simulink model "remoteMicrogrid"  (R2023a)
settings: Solver=FixedStepDiscrete  StartTime=0.0  StopTime=8  FixedStep=Ts  RelTol=1e-3
PreLoadFcn:
  | remoteMicrogridInputData
undefined symbols (not defined in the file): BESS, ControlRoom, DiscIntNeverNeededParam, Grid, Load, Machine, Microgrid, PV, T_on, Ts
libraries: ee_lib x46, eeGeneralControl x35, nesl_utility_internal x25, simulink x24, nesl_utility x20, fl_lib x17, slpidlib x12, eeTransforms x5, eeRmsMeasurement x4, eeTotalHarmonicDistorsion x4, eeSinusoidalMeasurement x3, batteryecm_lib x2
(part 2 of 5)

== system remoteMicrogrid/Diesel Substation, BESS, & Microgrid Controller/Diesel Generator ==
  AVR and Exciter : Subsystem
  "Governor and Prime Mover " : Subsystem  mask(Governor and Prime Mover){pu_speed_reference=Machine.SpeedReference, droop_percentage=Machine.Droop, pu_load_reference_setpoint=Machine.LoadReference, T_G=Machine.TimeConstandGovernor, T_CH=Machine.TimeConstantPrimeMover, base_torque=Machine.BaseTorque, pu_torque0=Machine.InitialTorque}
      mask prompts: pu_speed_reference "Speed reference, (pu)"; droop_percentage "Percentage droop, (%)"; pu_load_reference_setpoint "Load reference setpoint, (pu)"; T_G "Time constant of governor, (s)"; T_CH "Time constant of main inlet volumes and steam chest, (s)"; base_torque "Base torque, (N*m)"; pu_torque0 "Initial torque, (pu)"
      mask help:
      | Implements a synchronous machine governor and prime mover. The prime mover is a non-reheat steam turbine.
      |
      | The input to the block is a per-unit synchronous machine measurement vector.
      |
      | R and C are mechanical rotational ports.
  Machine Inertia : ee_lib/Electromechanical/Mechanical/Machine Inertia  SRated=Grid.DieselRatedPower V*A  FRated=Grid.Frequency Hz  nPolePairs=1  inertia_option=1  J=Machine.Inertia kg*m^2  H=3.525 s*W/V/A  damper_option=2  D=39.0509 N*m/(rad/s)  pu_D=0.01  initialization_option=2  fMechanical0=60 Hz  fElectrical0=Grid.Frequency Hz
      settings: InternalSimscapePortConfiguration="{\"Bottom\":[],\"Left\":[{\"id\":\"R\",\"label\":\"R\",\"type\":\"foundation.mechanical.rotational.rotational\"}],\"Right\":[],\"Top\":[]}"
  Rotational Friction : fl_lib/Mechanical/Rotational Elements/Rotational Friction  brkwy_trq=1.1 N*m  brkwy_vel=0.1 rad/s  Col_trq=0.05 N*m  visc_coef=0.001 N*m*s/rad  w_specify=off  w_priority=None  w=0 rad/s  w_nominal_specify=off  w_nominal_unit=rad/s  w_nominal_value=1  t_specify=off  t_priority=None  t=0 N*m  t_nominal_specify=off  t_nominal_unit=N*m  t_nominal_value=1
  Synchronous Machine Round Rotor : ee_lib/Electromechanical/Synchronous/Synchronous Machine Round Rotor  port_option=ee.enum.threePhasePort.composite  SRated=Grid.DieselRatedPower A*V  VRated=Grid.Voltage V  FRated=Grid.Frequency Hz  nPolePairs=1  param_option=ee.enum.sm.parameterization.standard  fieldCircuitParameterization_option=ee.enum.sm.fieldparameterization.current  baseEfd=92.95 V  baseIfd=1300 A  zero_sequence=ee.enum.park.zerosequence.include  axes_param=ee.enum.rotorangle.daxis  Ladu=1.66  Laqu=1.61  L0=0.15  Ll=0.05  Ra=0.03  Lfd=0.165  Rfd=0.0006  L1d=0.1713  R1d=0.0284  L1q=0.7252  R1q=0.00619  L2q=0.125  R2q=0.02368  Xl=0.05  Xd=1.72  Xq=0.79  X0=0.06  Xdd=0.13  Xqd=0.17  Xddd=0.09  Xqdd=0.12  d_option=ee.enum.circuit.open  Td0d=0.75 s  Tdd=0.03 s  Td0dd=0.03 s  Tddd=0.008 s  q_option=ee.enum.circuit.open  Tq0d=0.6 s  Tqd=0.03 s  Tq0dd=0.02 s  Tqdd=0.008 s  saturation_option=ee.enum.saturation.exclude  saturation_ifd=[0, .48, .76, 1.38, 1.79]  saturation_Vag=[0, .8, 1.08, 1.31, 1.4]  initialization_option=ee.enum.sm.initialization.steadystate  source_type=ee.enum.sm.load_flow_source_type.Swing  Vmag0=Grid.Voltage V  Vang0=0 deg  Pt0=Grid.DieselRatedPower A*V  Qt0=0 A*V  minimum_pu=0.95  phase_search_range=[-inf, inf] deg  gmin=1e-6 S  connection_option=ee.enum.Connection.wye  num_q_dampers=2  rotor_offset=-pi / 2 rad  pu_psid_specify=off  pu_psid_priority=None  pu_psid=0  pu_psid_nominal_specify=off  pu_psid_nominal_unit=1  pu_psid_nominal_value=1  pu_psiq_specify=off  pu_psiq_priority=None  pu_psiq=0  pu_psiq_nominal_specify=off  pu_psiq_nominal_unit=1  pu_psiq_nominal_value=1  pu_psifd_specify=off  pu_psifd_priority=None  pu_psifd=0  pu_psifd_nominal_specify=off  pu_psifd_nominal_unit=1  pu_psifd_nominal_value=1  pu_psi1d_specify=off  pu_psi1d_priority=None  pu_psi1d=0  pu_psi1d_nominal_specify=off  pu_psi1d_nominal_unit=1  pu_psi1d_nominal_value=1  pu_psi1q_specify=off  pu_psi1q_priority=None  pu_psi1q=0  pu_psi1q_nominal_specify=off  pu_psi1q_nominal_unit=1  pu_psi1q_nominal_value=1  pu_psi2q_specify=off  pu_psi2q_priority=None  pu_psi2q=0  pu_psi2q_nominal_specify=off  pu_psi2q_nominal_unit=1  pu_psi2q_nominal_value=1  angular_position_diff_specify=off  angular_position_diff_priority=None  angular_position_diff=180 deg  angular_position_diff_nominal_specify=off  angular_position_diff_nominal_unit=deg  angular_position_diff_nominal_value=1  Tmeas=298.15 K  alpha=3.93e-3 1/K  stator_thermal_mass=100 J/K  rotor_thermal_mass=200 J/K  temperatureA_specify=off  temperatureA_priority=High  temperatureA=25 degC  temperatureA_nominal_specify=off  temperatureA_nominal_unit=degC  temperatureA_nominal_value=1  temperatureB_specify=off  temperatureB_priority=High  temperatureB=25 degC  temperatureB_nominal_specify=off  temperatureB_nominal_unit=degC  temperatureB_nominal_value=1  temperatureC_specify=off  temperatureC_priority=High  temperatureC=25 degC  temperatureC_nominal_specify=off  temperatureC_nominal_unit=degC  temperatureC_nominal_value=1  temperatureR_specify=off  temperatureR_priority=High  temperatureR=25 degC  temperatureR_nominal_specify=off  temperatureR_nominal_unit=degC  temperatureR_nominal_value=1
      settings: InternalSimscapePortConfiguration="{\"Bottom\":[],\"Left\":[{\"id\":\"fd_p\",\"label\":\"fd+\",\"type\":\"foundation.electrical.electrical\"},{\"id\":\"fd_n\",\"label\":\"fd-\",\"type\":\"foundation.electrical.electrical\"},{\"id\":\"R\",\"label\":\"R\",\"type\":\"foundation.mechanical.rotational.rotational\"},{\"id\":\"C\",\"label\":\"C\",\"type\":\"foundation.mechanical.rotational.rotational\"}],\"Right\":[{\"id\":\"pu_output\",\"label\":\"pu\",\"type\":\"output\"},{\"id\":\"N\",\"label\":\"~\",\"type\":\"foundation.electrical.three_phase\"},{\"id\":\"n\",\"label\":\"n\",\"type\":\"foundation.electrical.electrical\"}],\"Top\":[]}"
  ref : PMIOPort  Side=Left
  ~ : PMIOPort  Port=2  Side=Right
  connections:
  ~/RConn1 -- Synchronous Machine Round Rotor/RConn2
  AVR and Exciter/LConn1 -- "Governor and Prime Mover "/LConn1 -- Synchronous Machine Round Rotor/RConn1
  "Governor and Prime Mover "/RConn1 -- Machine Inertia/LConn1 -- Synchronous Machine Round Rotor/LConn3 -- Rotational Friction/LConn1
  Synchronous Machine Round Rotor/LConn1 -- AVR and Exciter/RConn1
  ref/RConn1 -- Synchronous Machine Round Rotor/LConn2 -- AVR and Exciter/RConn2 -- Synchronous Machine Round Rotor/RConn3
  Synchronous Machine Round Rotor/LConn4 -- "Governor and Prime Mover "/RConn2 -- Rotational Friction/RConn1

== system remoteMicrogrid/Diesel Substation, BESS, & Microgrid Controller/Microgrid Controller ==
  "mPCC " : Inport
  CntrlRmSubstation : Inport  Port=2
  BESS : Inport  Port=3
  Active and Reactive Power Reference : Subsystem  mask{UpperPRef=Microgrid.UpperPRef, LowerPRef=Microgrid.LowerPRef}
      mask prompts: UpperPRef "Microgrid upper limit of power reference"; LowerPRef "Microgrid lower limit of power reference"
  Breaker Control : Subsystem
  Bus Creator1 : BusCreator  Inputs=3
  Bus Creator2 : BusCreator  Inputs=2
  Frequency Reference : Subsystem  mask{Frequency=Grid.Frequency, IslandFrequency=Microgrid.IslandFrequency}
      mask prompts: Frequency "Grid frequency"; IslandFrequency "Island frequency"
  PLL : Subsystem  mask{GridPLLKp=Grid.PLL_Kp, GridPLLKi=Grid.PLL_Ki}
      mask prompts: GridPLLKp "Grid PLL Proportional Gain"; GridPLLKi "Grid PLL Integral Gain"
  Planned Island from Diesel : Subsystem
  Resynchronization to Diesel : Subsystem
  Simulink-PS Converter : nesl_utility_internal/Simulink-PS Converter  PhysicalDomain=network_engine_domain  SubClassName=ps_input  LeftPortType=input  RightPortType=output  PseudoPeriodic=off  Frequencies=[]  NoiseDistribution=none  NoiseParameters=[]  Unit=1  AffineConversion=off  FilteringAndDerivatives=provide  SimscapeFilterOrder=1  InputFilterTimeConstant=0.001  UdotUserProvided=0
  Voltage Reference : Subsystem  mask{IslandVoltage=Microgrid.IslandVoltage}
      mask prompts: IslandVoltage "Microgrid island voltage"
  cBreaker : PMIOPort  Side=Right
  Out Bus Element1 : Outport  PortName=BESSRef  Element=Frequency
  Out Bus Element2 : Outport  PortName=BESSRef  Element=Voltage
  Out Bus Element3 : Outport  PortName=BESSRef  Element=Power
  Out Bus Element4 : Outport  PortName=BESSRef  Element=BRK
  MGController : Outport  Port=2
  wires:
  Frequency Reference/1(f_Ref) -> Out Bus Element1/1
  Voltage Reference/1(VRef) -> Out Bus Element2/1
  CntrlRmSubstation/1 -> Resynchronization to Diesel/2(Control Room), Planned Island from Diesel/2(Control Room), Active and Reactive Power Reference/1(CntrlRmSubstation), Breaker Control/1(CntrlRmSubstation), Voltage Reference/1(CntrlRmSubstation), Frequency Reference/1(CntrlRmSubstation)
  "mPCC "/1 -> Bus Creator1/3, PLL/1("mPCC ")  "PCC"
  BESS/1 -> Resynchronization to Diesel/3(BESS)
  Bus Creator1/1 -> Planned Island from Diesel/1(mPCCPLL), Resynchronization to Diesel/1(mPCCPLL)  "PLL"
  PLL/1(Grid) -> Bus Creator1/1  "Grid"
  PLL/2(Island) -> Bus Creator1/2  "Island"
  Planned Island from Diesel/1(IslandMGController) -> Bus Creator2/2
  Resynchronization to Diesel/1(ResynchMGController) -> Bus Creator2/1
  Bus Creator2/1 -> Voltage Reference/2(MGController), Frequency Reference/2(MGController), Breaker Control/2(MGController), Active and Reactive Power Reference/2(MGController), MGController/1  "MGController"
  Active and Reactive Power Reference/1(PQref) -> Out Bus Element3/1
  Breaker Control/1(BRK) -> Out Bus Element4/1, Simulink-PS Converter/1
  connections:
  cBreaker/RConn1 -- Simulink-PS Converter/RConn1

== system remoteMicrogrid/Diesel Substation, BESS, & Microgrid Controller/PCC Measurements and PCC Breaker ==
  Bus Creator : BusCreator  Inputs=2
  Circuit Breaker (Three-Phase) : ee_lib/Switches & Breakers/Circuit Breaker (Three-Phase)  R_closed=0.001 Ohm  G_open=1e-6 1/Ohm  threshold=0.5 V  breaker_behavior=ee.enum.switches.breakerBehavior.zeroCrossingDisable
      settings: InternalSimscapePortConfiguration="{\"Bottom\":[],\"Left\":[{\"id\":\"vT\",\"label\":\"vT\",\"type\":\"input\"},{\"id\":\"N1\",\"label\":\"~1\",\"type\":\"foundation.electrical.three_phase\"}],\"Right\":[{\"id\":\"N2\",\"label\":\"~2\",\"type\":\"foundation.electrical.three_phase\"}],\"Top\":[]}"
  Diesel Genset Current Measurement : Subsystem
  Diesel Genset Power Measurement : Subsystem
  ~ : PMIOPort  Side=Left
  "~ " : PMIOPort  Port=2  Side=Right
  cBreaker : PMIOPort  Port=3  Side=Right
  " mPCC" : Outport
  wires:
  Diesel Genset Current Measurement/1("Grid voltage ") -> Bus Creator/1  "Diesel voltage"
  Bus Creator/1 -> " mPCC"/1
  Diesel Genset Power Measurement/1(mPCC) -> Bus Creator/2  "mPCC"
  connections:
  Diesel Genset Current Measurement/RConn1 -- Circuit Breaker (Three-Phase)/LConn2
  Diesel Genset Power Measurement/RConn1 -- "~ "/RConn1
  cBreaker/RConn1 -- Circuit Breaker (Three-Phase)/LConn1
  Diesel Genset Power Measurement/LConn1 -- Circuit Breaker (Three-Phase)/RConn1
  ~/RConn1 -- Diesel Genset Current Measurement/LConn1

== system remoteMicrogrid/Diesel Substation, BESS, & Microgrid Controller/Transformer and Disconnectors ==
  Connectors : ee_lib/Passive/RLC Assemblies/RLC (Three-Phase)  component_structure=ee.enum.rlc.structure.R  R=Grid.ConnectorResistance Ohm  L=0.01 H  C=1e-6 F  R_parasitic=1e-6 Ohm  G_parasitic=1e-6 1/Ohm  IL_specify=on  IL_priority=High  IL=[0, 0, 0] A  IL_nominal_specify=off  IL_nominal_unit=A  IL_nominal_value=1  VC_specify=off  VC_priority=High  VC=[0, 0, 0] V  VC_nominal_specify=off  VC_nominal_unit=V  VC_nominal_value=1
      settings: InternalSimscapePortConfiguration="{\"Bottom\":[],\"Left\":[{\"id\":\"N1\",\"label\":\"~1\",\"type\":\"foundation.electrical.three_phase\"}],\"Right\":[{\"id\":\"N2\",\"label\":\"~2\",\"type\":\"foundation.electrical.three_phase\"}],\"Top\":[]}"
  Electrical Reference5 : fl_lib/Electrical/Electrical Elements/Electrical Reference
  Switchable 20 kW 4160 Vrms 60 Hz1 : ee_lib/Passive/RLC Assemblies/Wye-Connected Load  parameterization=ee.enum.rlc.parameterization.ratedpower  component_structure=ee.enum.rlc.structure.C  component_structure_PQ=ee.enum.rlc.structure.R  R=1 Ohm  L=0.001 H  C=1e-6 F  VRated=Microgrid.Voltage V  FRated=Grid.Frequency Hz  P=20000 W  Qpos=0 A*V  Qneg=-30000 A*V  R_parasitic=1e-6 Ohm  G_parasitic=1e-6 1/Ohm  R_parasitic_PQ=1e-6 Ohm  G_parasitic_PQ=1e-6 1/Ohm  Vmag0=Microgrid.Voltage V  Vang0=0 deg  Freq0=Microgrid.Frequency Hz  IL_specify=on  IL_priority=High  IL=[ 0 0 0 ] A  IL_nominal_specify=off  IL_nominal_unit=A  IL_nominal_value=1  VC_specify=on  VC_priority=High  VC=[ 0 0 0 ] V  VC_nominal_specify=off  VC_nominal_unit=V  VC_nominal_value=1
  Two-Winding Transformer (Three-Phase)1 : ee_lib/Passive/Transformers/Two-Winding Transformer (Three-Phase)  SRated=Grid.TransformerRating A*V  FRated=Grid.Frequency Hz  Winding1Connection=ee.enum.windingconnection.Y  VRated1=Grid.TransformerPrimaryVoltage V  Winding2Connection=ee.enum.windingconnection.Y  VRated2=Grid.TransformerSecondaryVoltage V  CoreType=ee.enum.coretype.threelimb  pu_Rw1=Grid.Primaryresistance  pu_Rw2=Grid.Secondaryresistance  leakage_reactance_option=ee.enum.transformer_leakage.include  pu_Xl1=Grid.Primaryreactance  pu_Xl2=Grid.Secondaryreactance  magnetizing_resistance_option=ee.enum.transformer_magnetizingResistance.include  pu_Rm=500  magnetizing_reactance_option=ee.enum.transformer_magnetizingReactance.include  saturation_option=ee.enum.transformer_saturation.exclude  pu_Xm=500  current_data=[0, .002, 1, 2]  magnetic_flux_data=[0, 1.2, 1.5, 1.51]  pu_X0=0.5  i1_specify=on  i1_priority=None  i1=[0, 0, 0] A  i1_nominal_specify=off  i1_nominal_unit=A  i1_nominal_value=1  i2_specify=on  i2_priority=None  i2=[0, 0, 0] A  i2_nominal_specify=off  i2_nominal_unit=A  i2_nominal_value=1  phi_specify=off  phi_priority=None  phi=[0, 0, 0]  phi_nominal_specify=off  phi_nominal_unit=1  phi_nominal_value=1  power_dissipated_specify=off  power_dissipated_priority=None  power_dissipated=0 W  power_dissipated_nominal_specify=off  power_dissipated_nominal_unit=W  power_dissipated_nominal_value=1
      settings: InternalSimscapePortConfiguration="{\"Bottom\":[],\"Left\":[{\"id\":\"N1\",\"label\":\"~1\",\"type\":\"foundation.electrical.three_phase\"}],\"Right\":[{\"id\":\"N2\",\"label\":\"~2\",\"type\":\"foundation.electrical.three_phase\"}],\"Top\":[]}"
  ~ : PMIOPort  Side=Left
  "~ " : PMIOPort  Port=2  Side=Right
  connections:
  Connectors/LConn1 -- Two-Winding Transformer (Three-Phase)1/RConn1
  Connectors/RConn1 -- Switchable 20 kW 4160 Vrms 60 Hz1/LConn1 -- "~ "/RConn1
  ~/RConn1 -- Two-Winding Transformer (Three-Phase)1/LConn1
  Switchable 20 kW 4160 Vrms 60 Hz1/RConn1 -- Electrical Reference5/LConn1

== system remoteMicrogrid/Feeder 2B & NO Switch/Subsystem ==
  ControlRoom : Inport
  Data Type Conversion : DataTypeConversion  SaturateOnIntegerOverflow=off  RndMeth=Floor
  Delay : Delay  DelayLength=6  SampleTime=0.15
  Logical Operator : Logic  Operator=NOT  AllPortsSameDT=off  OutDataTypeStr=boolean
  Simulink-PS Converter : nesl_utility/Simulink-PS Converter  PhysicalDomain=network_engine_domain  SubClassName=ps_input  LeftPortType=input  RightPortType=output  PseudoPeriodic=off  Frequencies=[]  NoiseDistribution=none  NoiseParameters=[]  Unit=1  AffineConversion=off  FilteringAndDerivatives=provide  SimscapeFilterOrder=1  InputFilterTimeConstant=0.001  UdotUserProvided=0
  Simulink-PS Converter1 : nesl_utility/Simulink-PS Converter  PhysicalDomain=network_engine_domain  SubClassName=ps_input  LeftPortType=input  RightPortType=output  PseudoPeriodic=off  Frequencies=[]  NoiseDistribution=none  NoiseParameters=[]  Unit=1  AffineConversion=off  FilteringAndDerivatives=provide  SimscapeFilterOrder=1  InputFilterTimeConstant=0.001  UdotUserProvided=0
  output1 : PMIOPort  Side=Right
  output : PMIOPort  Port=2  Side=Right
  wires:
  Logical Operator/1 -> Data Type Conversion/1
  ControlRoom/1 -> Logical Operator/1, Delay/1
  Data Type Conversion/1 -> Simulink-PS Converter/1
  Delay/1 -> Simulink-PS Converter1/1
  connections:
  Simulink-PS Converter/RConn1 -- output1/RConn1
  output/RConn1 -- Simulink-PS Converter1/RConn1

== system remoteMicrogrid/LV Load /Load Measurements1 ==
  Current and Voltage Sensor (Three-Phase)2 : ee_lib/Sensors & Transducers/Current and Voltage Sensor (Three-Phase)  vMeasurementType=ee.enum.vmeasurement.ll  outputUnit=ee.enum.unit.pu  SRated=150e3 A*V  VRated=Microgrid.LVVoltage V  I_specify=off  I_priority=None  I=[0, 0, 0] A  I_nominal_specify=off  I_nominal_unit=A  I_nominal_value=1  V_specify=off  V_priority=None  V=[0, 0, 0] V  V_nominal_specify=off  V_nominal_unit=V  V_nominal_value=1
      settings: InternalSimscapePortConfiguration="{\"Bottom\":[],\"Left\":[{\"id\":\"N1\",\"label\":\"~1\",\"type\":\"foundation.electrical.three_phase\"}],\"Right\":[{\"id\":\"V_output\",\"label\":\"V\",\"type\":\"output\"},{\"id\":\"I_output\",\"label\":\"I\",\"type\":\"output\"},{\"id\":\"N2\",\"label\":\"~2\",\"type\":\"foundation.electrical.three_phase\"}],\"Top\":[]}"
  Low-Pass Filter (Discrete or Continuous)1 : eeGeneralControl/Low-Pass Filter (Discrete or Continuous)  K=1  T=0.02  B=inf  A=-inf  init_option=Inherited from block input  x0=0  Ts=Ts
  Low-Pass Filter (Discrete or Continuous)2 : eeGeneralControl/Low-Pass Filter (Discrete or Continuous)  K=1  T=0.02  B=inf  A=-inf  init_option=Inherited from block input  x0=0  Ts=Ts
  PS-Simulink Converter : nesl_utility/PS-Simulink Converter  PhysicalDomain=network_engine_domain  SubClassName=ps_output  LeftPortType=input  RightPortType=output  PseudoPeriodic=off  Frequencies=[]  VectorFormat=inherit  Unit=inherit  AffineConversion=off
  PS-Simulink Converter1 : nesl_utility/PS-Simulink Converter  PhysicalDomain=network_engine_domain  SubClassName=ps_output  LeftPortType=input  RightPortType=output  PseudoPeriodic=off  Frequencies=[]  VectorFormat=inherit  Unit=inherit  AffineConversion=off
  PS-Simulink Converter12 : nesl_utility_internal/PS-Simulink Converter  PhysicalDomain=network_engine_domain  SubClassName=ps_output  LeftPortType=input  RightPortType=output  PseudoPeriodic=off  Frequencies=[]  VectorFormat=1-D array  Unit=V  AffineConversion=off
  PS-Simulink Converter13 : nesl_utility_internal/PS-Simulink Converter  PhysicalDomain=network_engine_domain  SubClassName=ps_output  LeftPortType=input  RightPortType=output  PseudoPeriodic=off  Frequencies=[]  VectorFormat=1-D array  Unit=A  AffineConversion=off
  PS-Simulink Converter6 : nesl_utility_internal/PS-Simulink Converter  PhysicalDomain=network_engine_domain  SubClassName=ps_output  LeftPortType=input  RightPortType=output  PseudoPeriodic=off  Frequencies=[]  VectorFormat=1-D array  Unit=kW  AffineConversion=off
  PS-Simulink Converter7 : nesl_utility_internal/PS-Simulink Converter  PhysicalDomain=network_engine_domain  SubClassName=ps_output  LeftPortType=input  RightPortType=output  PseudoPeriodic=off  Frequencies=[]  VectorFormat=1-D array  Unit=kV*A  AffineConversion=off
  Power Sensor (Three-Phase)1 : ee_lib/Sensors & Transducers/Power Sensor (Three-Phase)  load_type=ee.enum.passive.type_balanced.balanced  f0=60 Hz  config=ee.enum.with_neutral.no  rho=1
      settings: InternalSimscapePortConfiguration="{\"Bottom\":[],\"Left\":[{\"id\":\"N1\",\"label\":\"~1\",\"type\":\"foundation.electrical.three_phase\"}],\"Right\":[{\"id\":\"N2\",\"label\":\"~2\",\"type\":\"foundation.electrical.three_phase\"}],\"Top\":[{\"id\":\"Pm\",\"label\":\"P\",\"type\":\"output\"},{\"id\":\"Qm\",\"label\":\"Q\",\"type\":\"output\"}]}"
  RMS Measurement : eeRmsMeasurement/RMS Measurement  LabelModeActiveChoice=Total  F=Grid.Frequency  SpecifyHarmonics=off  K=[0 1 2]  Ts=Ts
      settings: LibrarySourceBlock=|
      | ee_sl_lib/Measurements/RMS
      | Measurement
  RMS Measurement1 : eeRmsMeasurement/RMS Measurement  LabelModeActiveChoice=Total  F=Grid.Frequency  SpecifyHarmonics=off  K=[0 1 2]  Ts=Ts
      settings: LibrarySourceBlock=|
      | ee_sl_lib/Measurements/RMS
      | Measurement
  "~ " : PMIOPort  Side=Left
  " ~ " : PMIOPort  Port=2  Side=Right
  Out Bus Element : Outport  PortName=mLoadF2  Element=active powerF2
  Out Bus Element1 : Outport  PortName=mLoadF2  Element=reactive powerF2
  Out Bus Element2 : Outport  PortName=mLoadF2  Element=voltageF2
  Out Bus Element3 : Outport  PortName=mLoadF2  Element=currentF2
  Out Bus Element4 : Outport  PortName=mLoadF2  Element=voltageRMSF2
  Out Bus Element5 : Outport  PortName=mLoadF2  Element=currentRMSF2
  wires:
  Low-Pass Filter (Discrete or Continuous)2/1 -> Out Bus Element1/1
  Low-Pass Filter (Discrete or Continuous)1/1 -> Out Bus Element/1
  PS-Simulink Converter6/1 -> Low-Pass Filter (Discrete or Continuous)1/1
  PS-Simulink Converter7/1 -> Low-Pass Filter (Discrete or Continuous)2/1
  PS-Simulink Converter13/1 -> Out Bus Element3/1
  PS-Simulink Converter12/1 -> Out Bus Element2/1
  PS-Simulink Converter/1 -> RMS Measurement/1
  RMS Measurement/1 -> Out Bus Element4/1
  RMS Measurement1/1 -> Out Bus Element5/1
  PS-Simulink Converter1/1 -> RMS Measurement1/1
  connections:
  Power Sensor (Three-Phase)1/RConn1 -- Current and Voltage Sensor (Three-Phase)2/LConn1
  Current and Voltage Sensor (Three-Phase)2/RConn1 -- PS-Simulink Converter/LConn1 -- PS-Simulink Converter12/LConn1
  Current and Voltage Sensor (Three-Phase)2/RConn2 -- PS-Simulink Converter1/LConn1 -- PS-Simulink Converter13/LConn1
  "~ "/RConn1 -- Power Sensor (Three-Phase)1/LConn1
  Current and Voltage Sensor (Three-Phase)2/RConn3 -- " ~ "/RConn1
  Power Sensor (Three-Phase)1/LConn2 -- PS-Simulink Converter6/LConn1
  Power Sensor (Three-Phase)1/LConn3 -- PS-Simulink Converter7/LConn1

== system remoteMicrogrid/MV Load/Load Measurements1 ==
  Current and Voltage Sensor (Three-Phase)2 : ee_lib/Sensors & Transducers/Current and Voltage Sensor (Three-Phase)  vMeasurementType=ee.enum.vmeasurement.ll  outputUnit=ee.enum.unit.pu  SRated=150e3 A*V  VRated=Microgrid.Voltage V  I_specify=off  I_priority=None  I=[0, 0, 0] A  I_nominal_specify=off  I_nominal_unit=A  I_nominal_value=1  V_specify=off  V_priority=None  V=[0, 0, 0] V  V_nominal_specify=off  V_nominal_unit=V  V_nominal_value=1
      settings: InternalSimscapePortConfiguration="{\"Bottom\":[],\"Left\":[{\"id\":\"N1\",\"label\":\"~1\",\"type\":\"foundation.electrical.three_phase\"}],\"Right\":[{\"id\":\"V_output\",\"label\":\"V\",\"type\":\"output\"},{\"id\":\"I_output\",\"label\":\"I\",\"type\":\"output\"},{\"id\":\"N2\",\"label\":\"~2\",\"type\":\"foundation.electrical.three_phase\"}],\"Top\":[]}"
  Low-Pass Filter (Discrete or Continuous)1 : eeGeneralControl/Low-Pass Filter (Discrete or Continuous)  K=1  T=0.02  B=inf  A=-inf  init_option=Inherited from block input  x0=0  Ts=Ts
  Low-Pass Filter (Discrete or Continuous)2 : eeGeneralControl/Low-Pass Filter (Discrete or Continuous)  K=1  T=0.02  B=inf  A=-inf  init_option=Inherited from block input  x0=0  Ts=Ts
  PS-Simulink Converter : nesl_utility/PS-Simulink Converter  PhysicalDomain=network_engine_domain  SubClassName=ps_output  LeftPortType=input  RightPortType=output  PseudoPeriodic=off  Frequencies=[]  VectorFormat=inherit  Unit=inherit  AffineConversion=off
  PS-Simulink Converter1 : nesl_utility_internal/PS-Simulink Converter  PhysicalDomain=network_engine_domain  SubClassName=ps_output  LeftPortType=input  RightPortType=output  PseudoPeriodic=off  Frequencies=[]  VectorFormat=1-D array  Unit=inherit  AffineConversion=off
  PS-Simulink Converter3 : nesl_utility/PS-Simulink Converter  PhysicalDomain=network_engine_domain  SubClassName=ps_output  LeftPortType=input  RightPortType=output  PseudoPeriodic=off  Frequencies=[]  VectorFormat=inherit  Unit=inherit  AffineConversion=off
  PS-Simulink Converter4 : nesl_utility_internal/PS-Simulink Converter  PhysicalDomain=network_engine_domain  SubClassName=ps_output  LeftPortType=input  RightPortType=output  PseudoPeriodic=off  Frequencies=[]  VectorFormat=1-D array  Unit=inherit  AffineConversion=off
  PS-Simulink Converter6 : nesl_utility_internal/PS-Simulink Converter  PhysicalDomain=network_engine_domain  SubClassName=ps_output  LeftPortType=input  RightPortType=output  PseudoPeriodic=off  Frequencies=[]  VectorFormat=1-D array  Unit=kW  AffineConversion=off
  PS-Simulink Converter7 : nesl_utility_internal/PS-Simulink Converter  PhysicalDomain=network_engine_domain  SubClassName=ps_output  LeftPortType=input  RightPortType=output  PseudoPeriodic=off  Frequencies=[]  VectorFormat=1-D array  Unit=kV*A  AffineConversion=off
  Power Sensor (Three-Phase)1 : ee_lib/Sensors & Transducers/Power Sensor (Three-Phase)  load_type=ee.enum.passive.type_balanced.balanced  f0=60 Hz  config=ee.enum.with_neutral.no  rho=1
      settings: InternalSimscapePortConfiguration="{\"Bottom\":[],\"Left\":[{\"id\":\"N1\",\"label\":\"~1\",\"type\":\"foundation.electrical.three_phase\"}],\"Right\":[{\"id\":\"N2\",\"label\":\"~2\",\"type\":\"foundation.electrical.three_phase\"}],\"Top\":[{\"id\":\"Pm\",\"label\":\"P\",\"type\":\"output\"},{\"id\":\"Qm\",\"label\":\"Q\",\"type\":\"output\"}]}"
  RMS Measurement : eeRmsMeasurement/RMS Measurement  LabelModeActiveChoice=Total  F=Grid.Frequency  SpecifyHarmonics=off  K=[0 1 2]  Ts=Ts
      settings: LibrarySourceBlock=|
      | ee_sl_lib/Measurements/RMS
      | Measurement
  RMS Measurement1 : eeRmsMeasurement/RMS Measurement  LabelModeActiveChoice=Total  F=Grid.Frequency  SpecifyHarmonics=off  K=[0 1 2]  Ts=Ts
      settings: LibrarySourceBlock=|
      | ee_sl_lib/Measurements/RMS
      | Measurement
  ~ : PMIOPort  Side=Left
  " ~ " : PMIOPort  Port=2  Side=Right
  Out Bus Element : Outport  PortName=mLoad  Element=active power
  Out Bus Element1 : Outport  PortName=mLoad  Element=reactive power
  Out Bus Element2 : Outport  PortName=mLoad  Element=voltage
  Out Bus Element3 : Outport  PortName=mLoad  Element=current
  Out Bus Element4 : Outport  PortName=mLoad  Element=voltageRMS
  Out Bus Element5 : Outport  PortName=mLoad  Element=currentRMS
  wires:
  PS-Simulink Converter7/1 -> Low-Pass Filter (Discrete or Continuous)2/1
  PS-Simulink Converter6/1 -> Low-Pass Filter (Discrete or Continuous)1/1
  Low-Pass Filter (Discrete or Continuous)1/1 -> Out Bus Element/1
  Low-Pass Filter (Discrete or Continuous)2/1 -> Out Bus Element1/1
  PS-Simulink Converter1/1 -> Out Bus Element2/1
  PS-Simulink Converter4/1 -> Out Bus Element3/1
  PS-Simulink Converter/1 -> RMS Measurement/1
  RMS Measurement/1 -> Out Bus Element5/1
  RMS Measurement1/1 -> Out Bus Element4/1
  PS-Simulink Converter3/1 -> RMS Measurement1/1
  connections:
  Power Sensor (Three-Phase)1/LConn3 -- PS-Simulink Converter7/LConn1
  Power Sensor (Three-Phase)1/LConn2 -- PS-Simulink Converter6/LConn1
  Current and Voltage Sensor (Three-Phase)2/RConn3 -- " ~ "/RConn1
  ~/RConn1 -- Power Sensor (Three-Phase)1/LConn1
  PS-Simulink Converter/LConn1 -- Current and Voltage Sensor (Three-Phase)2/RConn2 -- PS-Simulink Converter4/LConn1
  PS-Simulink Converter1/LConn1 -- PS-Simulink Converter3/LConn1 -- Current and Voltage Sensor (Three-Phase)2/RConn1
  Power Sensor (Three-Phase)1/RConn1 -- Current and Voltage Sensor (Three-Phase)2/LConn1

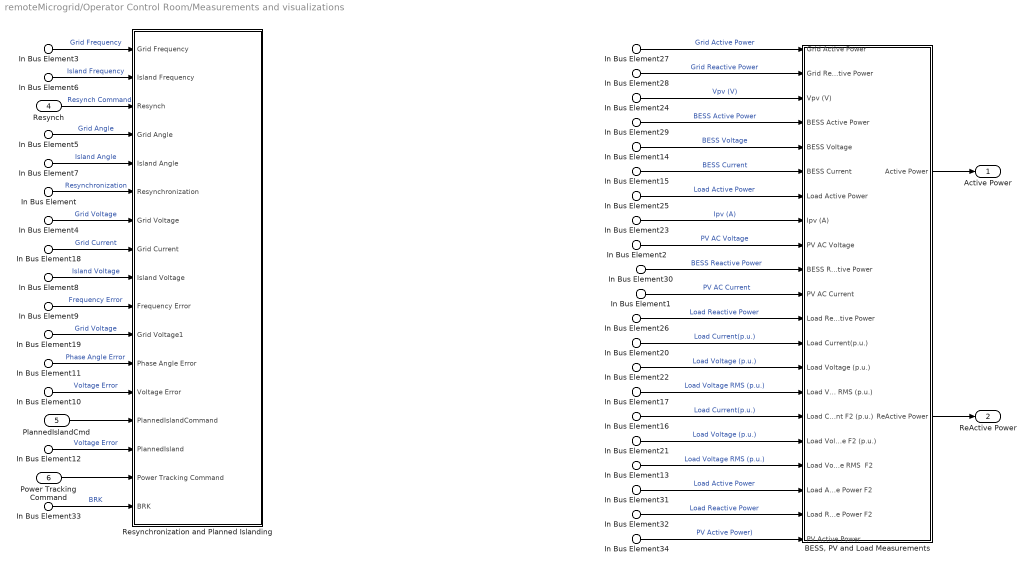
== system remoteMicrogrid/Operator Control Room/Measurements and visualizations  ==
  In Bus Element25 : Inport  PortName=mLoad  Element=active power
  In Bus Element17 : Inport  PortName=mLoad  Element=voltageRMS
  In Bus Element20 : Inport  PortName=mLoad  Element=current
  In Bus Element26 : Inport  PortName=mLoad  Element=reactive power
  In Bus Element22 : Inport  PortName=mLoad  Element=voltage
  In Bus Element4 : Inport  Port=2  PortName=MGController  Element=Controller.ResynchMGController.PCC measurments.Grid.voltage
  In Bus Element5 : Inport  Port=2  PortName=MGController  Element=Controller.ResynchMGController.PCC measurments.Grid.angle
  In Bus Element3 : Inport  Port=2  PortName=MGController  Element=Controller.ResynchMGController.PCC measurments.Grid.frequency
  In Bus Element8 : Inport  Port=2  PortName=MGController  Element=Controller.ResynchMGController.PCC measurments.Island.voltage
  In Bus Element7 : Inport  Port=2  PortName=MGController  Element=Controller.ResynchMGController.PCC measurments.Island.angle
  In Bus Element6 : Inport  Port=2  PortName=MGController  Element=Controller.ResynchMGController.PCC measurments.Island.frequency
  In Bus Element18 : Inport  Port=2  PortName=MGController  Element=Controller.ResynchMGController.PCC measurments.PCC.mPCC.current
  In Bus Element19 : Inport  Port=2  PortName=MGController  Element=Controller.ResynchMGController.PCC measurments.PCC.mPCC.voltage
  In Bus Element27 : Inport  Port=2  PortName=MGController  Element=Controller.ResynchMGController.PCC measurments.PCC.mPCC.activepower
  In Bus Element28 : Inport  Port=2  PortName=MGController  Element=Controller.ResynchMGController.PCC measurments.PCC.mPCC.reactivepower
  In Bus Element10 : Inport  Port=2  PortName=MGController  Element=Controller.ResynchMGController.MGResynch.voltagemagerror
  In Bus Element11 : Inport  Port=2  PortName=MGController  Element=Controller.ResynchMGController.MGResynch.phaseerror
  In Bus Element9 : Inport  Port=2  PortName=MGController  Element=Controller.ResynchMGController.MGResynch.frequencyerror
  In Bus Element : Inport  Port=2  PortName=MGController  Element=Controller.ResynchMGController.MGResynch.resynch
  In Bus Element12 : Inport  Port=2  PortName=MGController  Element=Controller.IslandMGController.MGPlannedIsland.plannedisland
  In Bus Element14 : Inport  Port=2  PortName=MGController  Element=BESS.voltage
  In Bus Element15 : Inport  Port=2  PortName=MGController  Element=BESS.current
  In Bus Element29 : Inport  Port=2  PortName=MGController  Element=BESS.active power
  In Bus Element30 : Inport  Port=2  PortName=MGController  Element=BESS.reactive power
  In Bus Element33 : Inport  Port=2  PortName=MGController  Element=References and BRK.BRK
  In Bus Element2 : Inport  Port=3  PortName=mPV  Element=PV ac.Va
  In Bus Element24 : Inport  Port=3  PortName=mPV  Element=PV ac.Va
  In Bus Element1 : Inport  Port=3  PortName=mPV  Element=PV ac.Ia
  In Bus Element23 : Inport  Port=3  PortName=mPV  Element=PV ac.Ia
  In Bus Element34 : Inport  Port=3  PortName=mPV  Element=PV power.PV active power
  Resynch : Inport  Port=4
  PlannedIslandCmd : Inport  Port=5
  Power Tracking Command : Inport  Port=6
  In Bus Element13 : Inport  Port=7  PortName=mLoadF2  Element=voltageRMSF2
  In Bus Element16 : Inport  Port=7  PortName=mLoadF2  Element=currentF2
  In Bus Element21 : Inport  Port=7  PortName=mLoadF2  Element=voltageF2
  In Bus Element31 : Inport  Port=7  PortName=mLoadF2  Element=active powerF2
  In Bus Element32 : Inport  Port=7  PortName=mLoadF2  Element=reactive powerF2
  "BESS, PV and Load Measurements" : Subsystem
  Resynchronization and Planned Islanding : Subsystem
  Active Power : Outport
  ReActive Power : Outport  Port=2
  wires:
  In Bus Element3/1 -> Resynchronization and Planned Islanding/1(Grid Frequency)  "Grid Frequency"
  In Bus Element6/1 -> Resynchronization and Planned Islanding/2(Island Frequency)  "Island Frequency"
  Resynch/1 -> Resynchronization and Planned Islanding/3(Resynch)  "Resynch Command"
  In Bus Element5/1 -> Resynchronization and Planned Islanding/4(Grid Angle)  "Grid Angle"
  In Bus Element7/1 -> Resynchronization and Planned Islanding/5(Island Angle)  "Island Angle"
  In Bus Element/1 -> Resynchronization and Planned Islanding/6(Resynchronization)  "Resynchronization"
  In Bus Element4/1 -> Resynchronization and Planned Islanding/7(Grid Voltage)  "Grid Voltage"
  In Bus Element18/1 -> Resynchronization and Planned Islanding/8(Grid Current)  "Grid Current"
  In Bus Element8/1 -> Resynchronization and Planned Islanding/9(Island Voltage)  "Island Voltage"
  In Bus Element9/1 -> Resynchronization and Planned Islanding/10(Frequency Error)  "Frequency Error"
  In Bus Element19/1 -> Resynchronization and Planned Islanding/11(Grid Voltage1)  "Grid Voltage"
  In Bus Element11/1 -> Resynchronization and Planned Islanding/12(Phase Angle Error)  "Phase Angle Error"
  In Bus Element10/1 -> Resynchronization and Planned Islanding/13(Voltage Error)  "Voltage Error"
  In Bus Element27/1 -> "BESS, PV and Load Measurements"/1(Grid Active Power)  "Grid Active Power"
  In Bus Element24/1 -> "BESS, PV and Load Measurements"/3(Vpv (V))  "Vpv (V)"
  In Bus Element15/1 -> "BESS, PV and Load Measurements"/6(BESS Current)  "BESS Current"
  In Bus Element25/1 -> "BESS, PV and Load Measurements"/7(Load Active Power)  "Load Active Power"
  In Bus Element23/1 -> "BESS, PV and Load Measurements"/8(Ipv (A))  "Ipv (A)"
  In Bus Element28/1 -> "BESS, PV and Load Measurements"/2(Grid Reactive Power)  "Grid Reactive Power"
  In Bus Element2/1 -> "BESS, PV and Load Measurements"/9(PV AC Voltage)  "PV AC Voltage"
  In Bus Element30/1 -> "BESS, PV and Load Measurements"/10(BESS Reactive Power)  "BESS Reactive Power"
  In Bus Element1/1 -> "BESS, PV and Load Measurements"/11(PV AC Current)  "PV AC Current"
  In Bus Element26/1 -> "BESS, PV and Load Measurements"/12(Load Reactive Power)  "Load Reactive Power"
  In Bus Element20/1 -> "BESS, PV and Load Measurements"/13(Load Current(p.u.))  "Load Current(p.u.)"
  In Bus Element22/1 -> "BESS, PV and Load Measurements"/14(Load Voltage (p.u.))  "Load Voltage (p.u.)"
  In Bus Element17/1 -> "BESS, PV and Load Measurements"/15(Load Voltage RMS (p.u.))  "Load Voltage RMS (p.u.)"
  In Bus Element29/1 -> "BESS, PV and Load Measurements"/4(BESS Active Power)  "BESS Active Power"
  In Bus Element14/1 -> "BESS, PV and Load Measurements"/5(BESS Voltage)  "BESS Voltage"
  PlannedIslandCmd/1 -> Resynchronization and Planned Islanding/14(PlannedIslandCommand)
  In Bus Element12/1 -> Resynchronization and Planned Islanding/15(PlannedIsland)  "Voltage Error"
  Power Tracking Command/1 -> Resynchronization and Planned Islanding/16(Power Tracking Command)
  In Bus Element13/1 -> "BESS, PV and Load Measurements"/18(Load Voltage RMS  F2)  "Load Voltage RMS (p.u.)"
  In Bus Element21/1 -> "BESS, PV and Load Measurements"/17(Load Voltage F2 (p.u.))  "Load Voltage (p.u.)"
  In Bus Element16/1 -> "BESS, PV and Load Measurements"/16(Load Current F2 (p.u.))  "Load Current(p.u.)"
  In Bus Element31/1 -> "BESS, PV and Load Measurements"/19("Load Active Power F2 ")  "Load Active Power"
  In Bus Element32/1 -> "BESS, PV and Load Measurements"/20(Load Reactive Power F2)  "Load Reactive Power"
  In Bus Element33/1 -> Resynchronization and Planned Islanding/17(BRK)  "BRK"
  In Bus Element34/1 -> "BESS, PV and Load Measurements"/21(PV Active Power)  "PV Active Power)"
  "BESS, PV and Load Measurements"/1(Active Power) -> Active Power/1
  "BESS, PV and Load Measurements"/2(ReActive Power) -> ReActive Power/1

== system remoteMicrogrid/Operator Control Room/Monitoring of system performance ==
  Active and Reactive Power : Inport
  mLoadF2 : Inport  Port=2
  In Bus Element1 : Inport  Port=3  PortName=mLoad  Element=active power
  In Bus Element4 : Inport  Port=3  PortName=mLoad  Element=voltage
  In Bus Element5 : Inport  Port=3  PortName=mLoad  Element=voltageRMS
  In Bus Element7 : Inport  Port=3  PortName=mLoad  Element=current
  In Bus Element9 : Inport  Port=3  PortName=mLoad  Element=currentRMS
  In Bus Element10 : Inport  Port=4  PortName=MGController  Element=Controller.IslandMGController.PCC measurments.PCC.mPCC.current
  In Bus Element6 : Inport  Port=4  PortName=MGController  Element=Controller.ResynchMGController.PCC measurments.Island.frequency
  In Bus Element8 : Inport  Port=4  PortName=MGController  Element=Controller.ResynchMGController.PCC measurments.Island.voltage
  In Bus Element2 : Inport  Port=4  PortName=MGController  Element=Controller.ResynchMGController.PCC measurments.PCC.mPCC.voltage
  "Load " : Subsystem
  Microgrid : Subsystem
  Subsystem : Subsystem
  THD : Subsystem
  wires:
  In Bus Element4/1 -> THD/1(mLoad)
  In Bus Element7/1 -> THD/2(In2)
  In Bus Element2/1 -> THD/3(MGController)
  In Bus Element10/1 -> THD/4(In4)
  In Bus Element6/1 -> Microgrid/1(In1)
  In Bus Element8/1 -> Microgrid/2(In2)
  In Bus Element5/1 -> "Load "/1(In1)
  In Bus Element9/1 -> "Load "/2(In2)
  In Bus Element1/1 -> "Load "/3(In3)
  Active and Reactive Power/1 -> Subsystem/1(Active and Reactive Power)
  mLoadF2/1 -> Subsystem/2(mLoadF2)

== system remoteMicrogrid/Operator Control Room/Power Tracking ==
  MGController : Inport
  In2 : Inport  Port=2
  Bus Selector : BusSelector  OutputSignals=References and BRK.BRK,Controller.ResynchMGController.MGResynch.resynch
  Delay : Delay  DelayLength=200  SampleTime=50*Ts
  Power Command : Step  Time=0.5  SampleTime=Ts
  Power Command1 : Step  Time=50  After=-1  SampleTime=Ts
  Sum : Sum  Inputs=|++
  Switch : Switch  Criteria=u2 > Threshold  Threshold=0.5  SaturateOnIntegerOverflow=off  InputSameDT=off
  Switch1 : Switch  Criteria=u2 > Threshold  Threshold=0.5  SaturateOnIntegerOverflow=off  InputSameDT=off
  Switch2 : Switch  Criteria=u2 > Threshold  Threshold=0.5  SaturateOnIntegerOverflow=off  InputSameDT=off
  Switchoff Power Tracking : Constant  Value=0
  Switchoff Power Tracking1 : Constant  Value=0
  Switchoff Power Tracking3 : Constant
  Power tracking off : Outport
  wires:
  Switchoff Power Tracking/1 -> Switch/1  "Power tracking off"
  Bus Selector/1 -> Switch/2  "<BRK>"
  Delay/1 -> Switch2/2  "Resynch Delay"
  MGController/1 -> Bus Selector/1
  Sum/1 -> Switch/3  "Power tracking"
  Power Command1/1 -> Sum/2  "Power Tracking Command"
  Power Command/1 -> Sum/1  "Power Tracking Command"
  Bus Selector/2 -> Delay/1  "<resynch>"
  Switch2/1 -> Power tracking off/1  "Power tracking off"
  Switchoff Power Tracking3/1 -> Switch2/1  "Power tracking on"
  In2/1 -> Switch1/2  "ResynchCommand"
  Switch/1 -> Switch1/3  "PowerCmd"
  Switch1/1 -> Switch2/3  "PowerCmd"
  Switchoff Power Tracking1/1 -> Switch1/1  "Power tracking off"

== system remoteMicrogrid/PV /30 kW PV ==
  In Bus Element : Inport  PortName=PV
  Current and Voltage Sensor (Three-Phase)2 : ee_lib/Sensors & Transducers/Current and Voltage Sensor (Three-Phase)  vMeasurementType=ee.enum.vmeasurement.lg  outputUnit=ee.enum.unit.pu  SRated=PV.MVA_base_new A*V  VRated=PV.KV_base_new V  I_specify=off  I_priority=None  I=[0, 0, 0] A  I_nominal_specify=off  I_nominal_unit=A  I_nominal_value=1  V_specify=off  V_priority=None  V=[0, 0, 0] V  V_nominal_specify=off  V_nominal_unit=V  V_nominal_value=1
      settings: InternalSimscapePortConfiguration="{\"Bottom\":[],\"Left\":[{\"id\":\"N1\",\"label\":\"~1\",\"type\":\"foundation.electrical.three_phase\"}],\"Right\":[{\"id\":\"V_output\",\"label\":\"V\",\"type\":\"output\"},{\"id\":\"I_output\",\"label\":\"I\",\"type\":\"output\"},{\"id\":\"N2\",\"label\":\"~2\",\"type\":\"foundation.electrical.three_phase\"}],\"Top\":[]}"
  L Filter1 : Subsystem
  Measurement1 : Subsystem
  PS-Simulink Converter1 : nesl_utility/PS-Simulink Converter  PhysicalDomain=network_engine_domain  SubClassName=ps_output  LeftPortType=input  RightPortType=output  PseudoPeriodic=off  Frequencies=[]  VectorFormat=inherit  Unit=inherit  AffineConversion=off
  PS-Simulink Converter3 : nesl_utility/PS-Simulink Converter  PhysicalDomain=network_engine_domain  SubClassName=ps_output  LeftPortType=input  RightPortType=output  PseudoPeriodic=off  Frequencies=[]  VectorFormat=inherit  Unit=inherit  AffineConversion=off
  PV Inverter 2 : Subsystem
  Terminator : Terminator
  ~ : PMIOPort  Side=Left
  PV power : Outport
  wires:
  PS-Simulink Converter3/1 -> Terminator/1
  PS-Simulink Converter1/1 -> Measurement1/1(u)
  In Bus Element/1 -> PV Inverter 2/1(PV)
  Measurement1/1(ipv1) -> PV Inverter 2/2(ipv1)
  PV Inverter 2/1(PV power) -> PV power/1
  connections:
  L Filter1/RConn1 -- Current and Voltage Sensor (Three-Phase)2/LConn1
  PV Inverter 2/RConn1 -- L Filter1/LConn1
  PS-Simulink Converter3/LConn1 -- Current and Voltage Sensor (Three-Phase)2/RConn1
  PS-Simulink Converter1/LConn1 -- Current and Voltage Sensor (Three-Phase)2/RConn2
  ~/RConn1 -- Current and Voltage Sensor (Three-Phase)2/RConn3

== system remoteMicrogrid/PV /PLL & Measurements ==
  V : Inport
  Measurement2 : Subsystem
  Subsystem : Subsystem
  Out Bus Element : Outport  PortName=PV  Element=Vq
  Out Bus Element1 : Outport  PortName=PV  Element=Vd
  Out Bus Element2 : Outport  PortName=PV  Element=w
  Out Bus Element3 : Outport  PortName=PV  Element=Theta
  Out Bus Element4 : Outport  PortName=PV  Element=Vmag
  wires:
  V/1 -> Measurement2/1(u)
  Subsystem/2(freq) -> Out Bus Element2/1
  Subsystem/5(Vq) -> Out Bus Element/1
  Subsystem/3(angle) -> Out Bus Element3/1
  Subsystem/4(Vd) -> Out Bus Element1/1
  Measurement2/1(Vg) -> Subsystem/1(abc)
  Subsystem/1(mag) -> Out Bus Element4/1

== system remoteMicrogrid/Selected Results/Inverter Active & Reactive Power  ==
  Vabc : Inport
  Iabc : Inport  Port=2
  Demux : Demux  Outputs=3
  Gain : Gain  Gain=1/sqrt(3)
  Low-Pass Filter (Discrete or Continuous) : eeGeneralControl/Low-Pass Filter (Discrete or Continuous)  K=1  T=0.02  B=inf  A=-inf  init_option=Inherited from block input  x0=0  Ts=-1
  Low-Pass Filter (Discrete or Continuous)1 : eeGeneralControl/Low-Pass Filter (Discrete or Continuous)  K=1  T=0.02  B=inf  A=-inf  init_option=Inherited from block input  x0=0  Ts=-1
  Minus : Sum  Inputs=+-
  Minus1 : Sum  Inputs=+-
  Minus2 : Sum  Inputs=+-
  Mux : Mux  Inputs=3
  Product : Product
  Product1 : Product
  Sum of Elements : Sum  Inputs=+
  Sum of Elements1 : Sum  Inputs=+
  gain : Gain  Gain=2/3
  gain1 : Gain  Gain=2/3
  P : Outport  VectorParamsAs1DForOutWhenUnconnected=off
  Q : Outport  Port=2  VectorParamsAs1DForOutWhenUnconnected=off
  wires:
  Minus/1 -> Mux/3
  Minus2/1 -> Mux/2
  Minus1/1 -> Mux/1
  Gain/1 -> Low-Pass Filter (Discrete or Continuous)1/1
  Sum of Elements1/1 -> Gain/1
  Product1/1 -> Sum of Elements1/1
  Mux/1 -> Product1/2
  Demux/3 -> Minus1/2, Minus2/1
  Demux/2 -> Minus/2, Minus1/1
  Demux/1 -> Minus/1, Minus2/2
  Sum of Elements/1 -> Low-Pass Filter (Discrete or Continuous)/1
  Product/1 -> Sum of Elements/1
  Iabc/1 -> Product/2, Product1/1
  Vabc/1 -> Product/1, Demux/1
  Low-Pass Filter (Discrete or Continuous)/1 -> gain/1
  Low-Pass Filter (Discrete or Continuous)1/1 -> gain1/1
  gain/1 -> P/1  "BESS Active Power(pu)"
  gain1/1 -> Q/1  "BESS Reactive Power(pu)"

== system remoteMicrogrid/Diesel Substation, BESS, & Microgrid Controller/BESS and Controller/BESS ==
  Average-Value Voltage Source Converter (Three-Phase) : ee_lib/Semiconductors & Converters/Converters/Average-Value Voltage Source Converter (Three-Phase)  port_option=ee.enum.threePhasePort.expanded  frequency_option=ee.enum.converters.frequency.variable  FRated=60 Hz  losses_parameterization=ee.enum.converters.losses.fixed  Pfixed=1 W  ks=0.01  kc1=1.7 V  kc2=0.01 Ohm  Ploss_vect=[100, 800, 1870, 3250, 4900] W  Irms_vect=[10, 100, 200, 300, 400] A  Vdc_nom=300 V  thermal_mass=30000 J/K  temperature_specify=off  temperature_priority=High  temperature=298.15 K  temperature_nominal_specify=off  temperature_nominal_unit=K  temperature_nominal_value=1
      settings: InternalSimscapePortConfiguration="{\"Bottom\":[],\"Left\":[{\"id\":\"ModWave\",\"label\":\"ModWave\",\"type\":\"input\"},{\"id\":\"a\",\"label\":\"a\",\"type\":\"foundation.electrical.electrical\"},{\"id\":\"b\",\"label\":\"b\",\"type\":\"foundation.electrical.electrical\"},{\"id\":\"c\",\"label\":\"c\",\"type\":\"foundation.electrical.electrical\"}],\"Right\":[{\"id\":\"p\",\"label\":\"+\",\"type\":\"foundation.electrical.electrical\"},{\"id\":\"n\",\"label\":\"-\",\"type\":\"foundation.electrical.electrical\"}],\"Top\":[]}"
  Battery : batteryecm_lib/Battery  Vnom=BESS.Vdc V  prm_dir=simscape.enum.battery.prm_dir.disabled  R1_dis=2 Ohm  R1_ch=2 Ohm  R1=BESS.Rs Ohm  prm_AH=simscape.enum.battery.prm_AH.infinite  AH=50 A*hr  V1=11.5 V  AH1=25 A*hr  prm_R2=simscape.enum.battery.prm_R2.disabled  R2=2000 Ohm  Tmeas=298.15 K  charge_measurement_port=simscape.enum.battery.enable.no  prm_dyn=simscape.enum.battery.prm_dyn.off  Rp1=0.005 Ohm  tau1=30 s  Rp2=0.005 Ohm  tau2=30 s  Rp3=0.005 Ohm  tau3=30 s  Rp4=0.005 Ohm  tau4=30 s  Rp5=0.005 Ohm  tau5=30 s  prm_fade=simscape.enum.battery.prm_fade.disabled  N_fade=100  AH_fade=45 A*hr  R1_fade=2.02 Ohm  R1_ch_fade=2.02 Ohm  V1_fade=10.35 V  prm_age=simscape.enum.battery.prm_age.disabled  prm_age_OCV=simscape.enum.battery.prm_age_OCV.OCV  OCV_age=0.9  SOC_age=60  Tmeas_age=298.15 K  delta_time_age_vec=[0] d  temperature_age_vec=[273] K  OCV_scaling_age=2.2134e6  OCV_offset_age=1.632e6  temp_exp_age=0.515833569 V  t_exp_age=0.75  Vnom_T2=12 V  R1_T2=2.2 Ohm  R1_T2_dis=2.2 Ohm  R1_T2_ch=2.2 Ohm  V1_T2=11.4 V  R2_T2=2200 Ohm  Rp1_T2=0.005 Ohm  tau1_T2=30 s  Rp2_T2=0.005 Ohm  tau2_T2=30 s  Rp3_T2=0.005 Ohm  tau3_T2=30 s  Rp4_T2=0.005 Ohm  tau4_T2=30 s  Rp5_T2=0.005 Ohm  tau5_T2=30 s  Tmeas2=273.15 K  thermal_port=simscape.enum.thermaleffects.omit  thermal_mass=30000 J/K  i_specify=off  i_priority=None  i=0 A  i_nominal_specify=off  i_nominal_unit=A  i_nominal_value=1  v_specify=off  v_priority=None  v=0 V  v_nominal_specify=off  v_nominal_unit=V  v_nominal_value=1  charge_specify=off  charge_priority=High  charge=50 A*hr  charge_nominal_specify=off  charge_nominal_unit=A*hr  charge_nominal_value=1  num_cycles_specify=off  num_cycles_priority=High  num_cycles=0  num_cycles_nominal_specify=off  num_cycles_nominal_unit=1  num_cycles_nominal_value=1  temperature_specify=off  temperature_priority=High  temperature=298.15 K  temperature_nominal_specify=off  temperature_nominal_unit=K  temperature_nominal_value=1
  Battery1 : batteryecm_lib/Battery  Vnom=BESS.Vdc V  prm_dir=simscape.enum.battery.prm_dir.disabled  R1_dis=2 Ohm  R1_ch=2 Ohm  R1=BESS.Rs Ohm  prm_AH=simscape.enum.battery.prm_AH.infinite  AH=50 A*hr  V1=11.5 V  AH1=25 A*hr  prm_R2=simscape.enum.battery.prm_R2.disabled  R2=2000 Ohm  Tmeas=298.15 K  charge_measurement_port=simscape.enum.battery.enable.no  prm_dyn=simscape.enum.battery.prm_dyn.off  Rp1=0.005 Ohm  tau1=30 s  Rp2=0.005 Ohm  tau2=30 s  Rp3=0.005 Ohm  tau3=30 s  Rp4=0.005 Ohm  tau4=30 s  Rp5=0.005 Ohm  tau5=30 s  prm_fade=simscape.enum.battery.prm_fade.disabled  N_fade=100  AH_fade=45 A*hr  R1_fade=2.02 Ohm  R1_ch_fade=2.02 Ohm  V1_fade=10.35 V  prm_age=simscape.enum.battery.prm_age.disabled  prm_age_OCV=simscape.enum.battery.prm_age_OCV.OCV  OCV_age=0.9  SOC_age=60  Tmeas_age=298.15 K  delta_time_age_vec=[0] d  temperature_age_vec=[273] K  OCV_scaling_age=2.2134e6  OCV_offset_age=1.632e6  temp_exp_age=0.515833569 V  t_exp_age=0.75  Vnom_T2=12 V  R1_T2=2.2 Ohm  R1_T2_dis=2.2 Ohm  R1_T2_ch=2.2 Ohm  V1_T2=11.4 V  R2_T2=2200 Ohm  Rp1_T2=0.005 Ohm  tau1_T2=30 s  Rp2_T2=0.005 Ohm  tau2_T2=30 s  Rp3_T2=0.005 Ohm  tau3_T2=30 s  Rp4_T2=0.005 Ohm  tau4_T2=30 s  Rp5_T2=0.005 Ohm  tau5_T2=30 s  Tmeas2=273.15 K  thermal_port=simscape.enum.thermaleffects.omit  thermal_mass=30000 J/K  i_specify=off  i_priority=None  i=0 A  i_nominal_specify=off  i_nominal_unit=A  i_nominal_value=1  v_specify=off  v_priority=None  v=0 V  v_nominal_specify=off  v_nominal_unit=V  v_nominal_value=1  charge_specify=off  charge_priority=High  charge=50 A*hr  charge_nominal_specify=off  charge_nominal_unit=A*hr  charge_nominal_value=1  num_cycles_specify=off  num_cycles_priority=High  num_cycles=0  num_cycles_nominal_specify=off  num_cycles_nominal_unit=1  num_cycles_nominal_value=1  temperature_specify=off  temperature_priority=High  temperature=298.15 K  temperature_nominal_specify=off  temperature_nominal_unit=K  temperature_nominal_value=1
  Electrical Reference4 : fl_lib/Electrical/Electrical Elements/Electrical Reference
  Phase Splitter : ee_lib/Connectors & References/Phase Splitter
  Modulation : PMIOPort  Side=Left
  ~ : PMIOPort  Port=2  Side=Left
  connections:
  Battery/LConn1 -- Average-Value Voltage Source Converter (Three-Phase)/RConn1
  Battery/RConn1 -- Battery1/LConn1 -- Electrical Reference4/LConn1
  Phase Splitter/RConn3 -- Average-Value Voltage Source Converter (Three-Phase)/LConn4
  Battery1/RConn1 -- Average-Value Voltage Source Converter (Three-Phase)/RConn2
  Phase Splitter/RConn1 -- Average-Value Voltage Source Converter (Three-Phase)/LConn2
  Modulation/RConn1 -- Average-Value Voltage Source Converter (Three-Phase)/LConn1
  Phase Splitter/RConn2 -- Average-Value Voltage Source Converter (Three-Phase)/LConn3
  Phase Splitter/LConn1 -- ~/RConn1
